simulink model "observer_SIMPLES"  (Simulink 8.5)
settings: Solver=ode45  StartTime=0.0  StopTime=T  RelTol=1e-5
values from neighbouring files (symbols this model uses):
  C = eye(5,5)    [Home.m]
  D = zeros(1,2)    [Home.m]    (also in analysis.m)
  K = lqr(A, B, Qr, Rr)    [Home.m]    (also in analysis.m; fp_ini.m)
  L = lqe(A, G, C, Qe, Re)    [Home.m]    (also in analysis.m; fp_ini.m)
  x0 = [alpha 0 beta 0 0]'    [Home.m]    (also in analysis.m)
undefined symbols (not defined in the file or in its folder): A, B
settings Model: Creator=João Pedro Belfo  LastModifiedBy=luisr
settings DataIOCC: SignalLoggingSaveFormat=Dataset
settings OptimizationCC: ExpressionDepthLimit=128
settings DebuggingCC: UnderspecifiedInitializationDetection=Simplified  MergeDetectMultiDrivingBlocksExec=error  FcnCallInpInsideContextMsg=EnableAllAsError  StateNameClashWarn=none
settings GRTTargetCC: CombineOutputUpdateFcns=on  GRTInterface=off

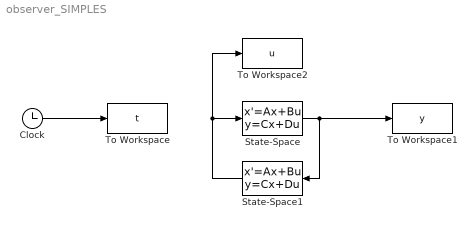
== system observer_SIMPLES ==
  Clock : Clock
  State-Space : StateSpace  A=A  B=B  C=C  D=[0;0]  X0=x0
  State-Space1 : StateSpace  A=A-B*K-L*C  B=L  C=-K  D=D  X0=0
  To Workspace : ToWorkspace  VariableName=t  SaveFormat=Timeseries  SampleTime=-1
  To Workspace1 : ToWorkspace  VariableName=y  SaveFormat=Timeseries  SampleTime=-1
  To Workspace2 : ToWorkspace  VariableName=u  SaveFormat=Timeseries  SampleTime=-1
  wires:
  Clock/1 -> To Workspace/1
  State-Space/1 -> State-Space1/1, To Workspace1/1
  State-Space1/1 -> To Workspace2/1, State-Space/1
